simulink model "template_seesaw_2018a"  (R2019b)
settings: Solver=ode45  StartTime=0.0  StopTime=10  FixedStep=0.005  RelTol=1e-3
values from neighbouring files (symbols this model uses):
  K = [66.2259572254 -60.3086645892 5.93307364323 -20.4157003719]    [lqr_K.mat]    (also in lqr_controller.m = lqr(sys,Q,R); swmain.m = lqr_controller(sys2))
  sys = ss(A,B,C,D,-1)    [1b.m]    (also in get_system.m = ss(A,B,C,D); get_system2.m = ss(A,B,C,D); statespace.m = ss(A,B,C,D); swmain.m = get_system(params))
  x_d = desired_state(theta_d, params)    [swmain.m]
undefined symbols (not defined in the file or in its folder): National_Instruments, PCI
libraries: sldrtlib x2, simulink_extras x1
settings Model: SimulationMode=external  ExtModeTrigDuration=200000  Creator=magudelo  LastModifiedBy=martijndebeuf
settings SolverCC: InsertRTBMode=Always
settings DataIOCC: LimitDataPoints=on  SaveFormat=Array  SignalLoggingSaveFormat=ModelDataLogs  ReturnWorkspaceOutputs=off
settings OptimizationCC: ExpressionDepthLimit=2147483647
settings DebuggingCC: UnderspecifiedInitializationDetection=Classic  MergeDetectMultiDrivingBlocksExec=none  SolverPrmCheckMsg=warning  FcnCallInpInsideContextMsg=warning  StateNameClashWarn=warning  SFUnexpectedBacktrackingDiag=warning  SFNoUnconditionalDefaultTransitionDiag=warning  SFExecutionAtInitializationDiag=none  ArithmeticOperatorsInVariantConditions=warning
settings ModelReferenceCC: PropagateSignalLabelsOutOfModel=off
settings SFSimCC: SimUseLocalCustomCode=off  CustomCodeUndefinedFunction=UseInterfaceOnly
settings RTWCC: Description=Simulink Desktop Real-Time  SystemTargetFile=sldrt.tlc  TemplateMakefile=sldrt.tmf  RTWUseLocalCustomCode=off  RTWCompilerOptimization=on
settings CodeAppCC: MaxIdLength=95  StateflowObjectComments=on
settings TargetCC: TargetPreCompLibLocation=C:\Program Files\MATLAB\R2018a\toolbox\sldrt\lib\win64  GeneratePreprocessorConditionals=Use local settings  PreserveStateflowLocalDataDimensions=off
settings ConfigComp: CovMetricSettings=dw  CovHtmlReporting=on  CovSaveCumulativeToWorkspaceVar=on  CovSaveSingleToWorkspaceVar=on  CovExternalEMLEnable=off

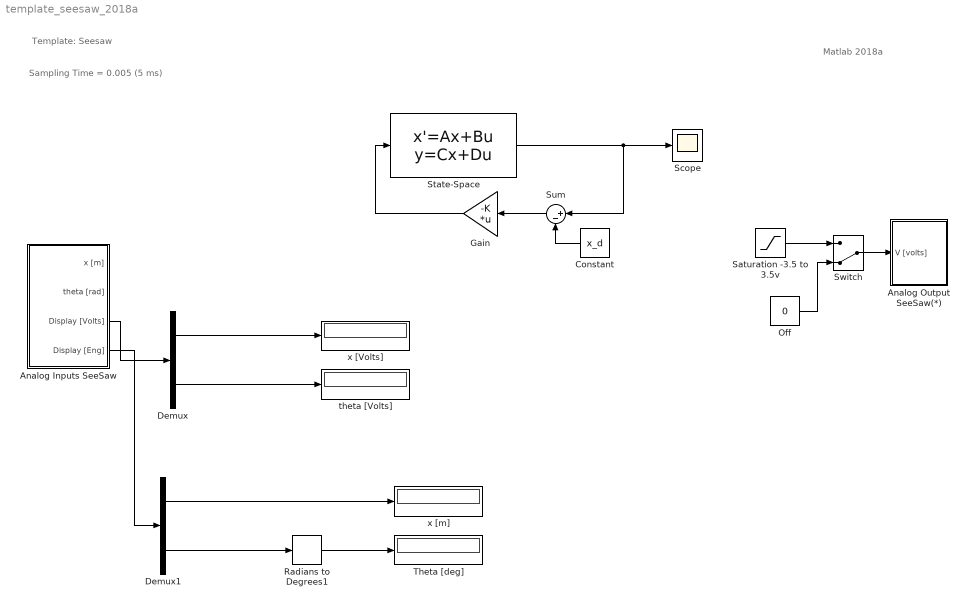
== system template_seesaw_2018a ==
  note: Matlab 2018a
  note: Template: Seesaw
  note: Sampling Time = 0.005 (5 ms)
  Analog Inputs SeeSaw : Subsystem  mask(Analog Inputs. SeeSaw){v2m=0.1033, offset_x=0, v2r=-0.0827, offset_theta=-5.56}
      mask prompts: v2m "F_x = Conversion factor from Volts to Meters:"; offset_x "Off_x = Offset for Cart Position [Volts] :"; v2r "F_theta = Conversion Factor From Volts to Radians :"; offset_theta "Off_theta = Offset for the angle of the SeeSaw [Volts] :"
      mask help:
      | Remember:
      |    Cart Position (x)                     => channel ACH0
      |    Angle of the SeeSaw (theta) => channel ACH1
      |
      |   Cart Position [m] = F_x *  ( Cart Position [v] + off_x )
      |   Angle of the SeeSaw [rad] = F_theta *  ( Angle of the SeeSaw [v] + off_theta )
  "Analog Output SeeSaw(*) " : Subsystem  mask(Analog Output - SeeSaw){}
      mask help:
      | Remember
      |    AO 0 => Power Amplifier + Motor
  Constant : Constant  Value=x_d
  Demux : Demux  Outputs=2
  Demux1 : Demux  Outputs=2
  Gain : Gain  Gain=-K  Multiplication=Matrix(K*u) (u vector)
  Off : Constant  Value=0
  Radians to Degrees1 : simulink_extras/Transformations/Radians to Degrees
  Saturation -3.5 to 3.5v : Saturate  UpperLimit=3.5  LowerLimit=-3.5
  Scope : Scope
  State-Space : StateSpace  A=sys.A  B=sys.B  C=eye(4)  D=zeros(4,1)  InitialCondition=initial_conditions'
  Sum : Sum  Inputs=|+-
  "Switch  " : ManualSwitch  CurrentSetting=0
  Theta [deg] : Display
      settings: SampleTime=0.25
  theta [Volts] : Display
      settings: SampleTime=0.25
  x [Volts] : Display
      settings: SampleTime=0.25
  x [m] : Display
      settings: SampleTime=0.25
  wires:
  Demux/1 -> x [Volts]/1
  Demux/2 -> theta [Volts]/1
  Analog Inputs SeeSaw/3(Display [Volts]) -> Demux/1
  Analog Inputs SeeSaw/4(Display [Eng]) -> Demux1/1
  Off/1 -> "Switch  "/2
  "Switch  "/1 -> "Analog Output SeeSaw(*) "/1(V [volts])
  Demux1/1 -> x [m]/1
  Demux1/2 -> Radians to Degrees1/1
  Radians to Degrees1/1 -> Theta [deg]/1
  Saturation -3.5 to 3.5v/1 -> "Switch  "/1
  State-Space/1 -> Sum/1, Scope/1
  Constant/1 -> Sum/2
  Sum/1 -> Gain/1
  Gain/1 -> State-Space/1

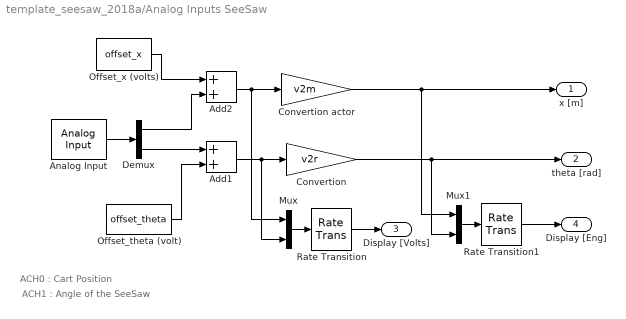
== system template_seesaw_2018a/Analog Inputs SeeSaw ==
  note: ACH0 : Cart Position
  note: ACH1 : Angle of the SeeSaw
  Add1 : Sum
  Add2 : Sum
  Analog Input : sldrtlib/Analog Input  SampleTime=0.005  MaxMissedTicks=10  ShowMissedTicks=off  YieldWhenWaiting=off  DrvName=National_Instruments/PCI-6014  DrvAddress=4294967295  DrvOptions=[1 0 0 0 0 0]  Channels=[1 2]  RangeMode=1  VoltRange=1  DataType=1
      settings: AttributesFormatString=National Instruments\nPCI-6014 [auto]  SourceProductName=Simulink Desktop Real-Time
  "Convertion " : Gain  Gain=v2r
  Convertion actor : Gain  Gain=v2m
  Demux : Demux  Outputs=2
  Mux : Mux  Inputs=2
  Mux1 : Mux  Inputs=2
  Offset_theta (volt) : Constant  Value=offset_theta
  Offset_x (volts) : Constant  Value=offset_x
  Rate Transition : RateTransition  OutPortSampleTime=0.25
  Rate Transition1 : RateTransition  OutPortSampleTime=0.25
  x [m] : Outport  VectorParamsAs1DForOutWhenUnconnected=off
  theta [rad] : Outport  Port=2  VectorParamsAs1DForOutWhenUnconnected=off
  Display [Volts] : Outport  Port=3  VectorParamsAs1DForOutWhenUnconnected=off
  Display [Eng] : Outport  Port=4  VectorParamsAs1DForOutWhenUnconnected=off
  wires:
  Analog Input/1 -> Demux/1
  Demux/1 -> Add2/2
  Add2/1 -> Convertion actor/1, Mux/1
  Offset_x (volts)/1 -> Add2/1
  Convertion actor/1 -> x [m]/1, Mux1/1
  Demux/2 -> Add1/1
  Offset_theta (volt)/1 -> Add1/2
  Add1/1 -> "Convertion "/1, Mux/2
  "Convertion "/1 -> theta [rad]/1, Mux1/2
  Rate Transition/1 -> Display [Volts]/1
  Mux/1 -> Rate Transition/1
  Mux1/1 -> Rate Transition1/1
  Rate Transition1/1 -> Display [Eng]/1

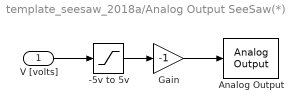
== system template_seesaw_2018a/Analog Output SeeSaw(*)  ==
  V [volts] : Inport
  -5v to 5v : Saturate  UpperLimit=5  LowerLimit=-5
  Analog Output : sldrtlib/Analog Output  SampleTime=0.005  MaxMissedTicks=10  ShowMissedTicks=off  YieldWhenWaiting=off  DrvName=National_Instruments/PCI-6014  DrvAddress=4294967295  DrvOptions=[1 0 0 0 0 0]  Channels=1  RangeMode=1  VoltRange=1  InitialValue=0  FinalValue=0
      settings: AttributesFormatString=National Instruments\nPCI-6014 [auto]  SourceProductName=Simulink Desktop Real-Time
  Gain : Gain  Gain=-1
  wires:
  Gain/1 -> Analog Output/1
  -5v to 5v/1 -> Gain/1
  V [volts]/1 -> -5v to 5v/1
